simulink model "microgrid_healthy_load_profiling_CDR_revD"  (Simulink 7.9)
settings: Solver=ode3  SolverMode=SingleTasking  StartTime=0.0  StopTime=12  FixedStep=1*10^(-4)  RelTol=1e-3
undefined symbols (not defined in the file): D1, Delta, tl1, tl2, tl3, tl4, tl5, tl6, Ts
libraries: powerlib x104, powerlib_extras x36
(part 1 of 2)
settings Model: Creator=SK  LastModifiedBy=SK
settings SolverCC: ZeroCrossAlgorithm=Adaptive  AlgebraicLoopSolver=LineSearch
settings OptimizationCC: SimCompilerOptimization=On  AccelVerboseBuild=on
settings SFSimCC: SFSimEnableDebug=off  SFSimEcho=off
settings RTWCC: RTWCompilerOptimization=On

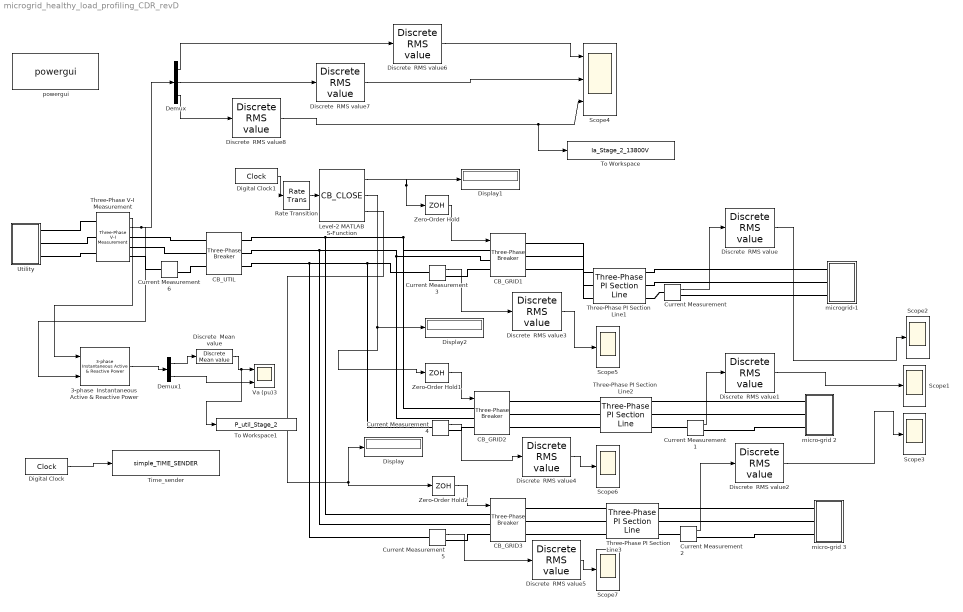
== system microgrid_healthy_load_profiling_CDR_revD ==
  3-phase  Instantaneous  Active & Reactive Power : powerlib_extras/Measurements/3-phase  Instantaneous  Active & Reactive Power
  CB_GRID1 : powerlib/Elements/Three-Phase Breaker  InitialState=closed  SwitchA=on  SwitchB=on  SwitchC=on  SwitchTimes="[4/60  10/60]"  External=on  BreakerResistance=0.001  SnubberResistance=1e6  SnubberCapacitance=inf  Measurements=None
  CB_GRID2 : powerlib/Elements/Three-Phase Breaker  InitialState=closed  SwitchA=on  SwitchB=on  SwitchC=on  SwitchTimes="[4/60  10/60]"  External=on  BreakerResistance=0.001  SnubberResistance=1e6  SnubberCapacitance=inf  Measurements=None
  CB_GRID3 : powerlib/Elements/Three-Phase Breaker  InitialState=closed  SwitchA=on  SwitchB=on  SwitchC=on  SwitchTimes="[4/60  10/60]"  External=on  BreakerResistance=0.001  SnubberResistance=1e6  SnubberCapacitance=inf  Measurements=None
  CB_UTIL : powerlib/Elements/Three-Phase Breaker  InitialState=closed  SwitchA=off  SwitchB=off  SwitchC=off  SwitchTimes="[4/60  10/60]"  External=off  BreakerResistance=0.001  SnubberResistance=1e6  SnubberCapacitance=inf  Measurements=None
  Current Measurement{,1..6} (7 alike) : powerlib/Measurements/Current Measurement  PhasorSimulation=off  OutputType=Complex  PSBequivalent=0
  Demux : Demux  Outputs=3
  Demux1 : Demux  Outputs=2
  Digital Clock : DigitalClock  SampleTime=Ts
  Digital Clock1 : DigitalClock  SampleTime=1e-4
  Discrete  Mean value : powerlib_extras/Discrete Measurements/Discrete  Mean value  Freq=60  Vinit=0  Ts=Ts
  Discrete  RMS value{,1..8} (9 alike) : powerlib_extras/Discrete Measurements/Discrete  RMS value  Freq=60  Mag_Init=0  Ts=Ts
  Display : Display
  Display1 : Display
  Display2 : Display
  Level-2 MATLAB S-Function : M-S-Function  FunctionName=CB_CLOSE
  Rate Transition : RateTransition
  Scope{1..3,5..7} (6 alike) : Scope
      Scope1 settings: YMin=0.95  YMax=1.05  SaveName=ScopeData3
      Scope2 settings: TimeRange=12  YMin=0  YMax=90
      Scope3 settings: YMin=0.95  YMax=1.05  SaveName=ScopeData4
      Scope5 settings: TimeRange=12  YMin=0  YMax=90  SaveName=ScopeData19
      Scope6 settings: TimeRange=12  YMin=0  YMax=90  SaveName=ScopeData20
      Scope7 settings: TimeRange=12  YMin=0  YMax=90  SaveName=ScopeData21
  Scope4 : Scope  NumInputPorts=3
      settings: TimeRange=12  YMin=54.0598~54.0598~54.0598  YMax=59.7504~59.7504~59.7504
  Three-Phase PI Section Line1 : powerlib/Elements/Three-Phase PI Section Line  LConnTagsString=a|b|c  RConnTagsString=A|B|C  Frequency=60  Resistances=[ 36.757 0.0]  Inductances="[ 0.126  0.0001]"  Capacitances=[0.00001 0.0001]  Length=2.06
  Three-Phase PI Section Line2 : powerlib/Elements/Three-Phase PI Section Line  LConnTagsString=a|b|c  RConnTagsString=A|B|C  Frequency=60  Resistances=[ 36.757 0.0]  Inductances="[ 0.126  0.0001]"  Capacitances=[0.00001 0.0001]  Length=2.06
  Three-Phase PI Section Line3 : powerlib/Elements/Three-Phase PI Section Line  LConnTagsString=a|b|c  RConnTagsString=A|B|C  Frequency=60  Resistances=[ 36.757 0.0]  Inductances="[ 0.126  0.0001]"  Capacitances=[0.00001 0.0001]  Length=2.06
  Three-Phase V-I Measurement : powerlib/Measurements/Three-Phase V-I Measurement  VoltageMeasurement=phase-to-ground  SetLabelV=off  LabelV=Vabc  Vpu=off  VpuLL=off  CurrentMeasurement=yes  SetLabelI=off  LabelI=Iabc  Ipu=off  Pbase=100e6  Vbase=500e3  OutputType=Magnitude  PhasorSimulation=off  PSBequivalent=0
  Time_sender : M-S-Function  FunctionName=simple_TIME_SENDER
  To Workspace : ToWorkspace  VariableName=Ia_Stage_2_13800V  SampleTime=5*Ts  SaveFormat=Structure With Time
  To Workspace1 : ToWorkspace  VariableName=P_util_Stage_2  SampleTime=5*Ts
  Utility : Subsystem
  Va (pu)3 : Scope  NumInputPorts=2
      settings: TickLabels=on  TimeRange=2  YMin=882000~-447440  YMax=974842~-447345  SaveName=vf
  Zero-Order Hold : ZeroOrderHold  SampleTime=0.3
  Zero-Order Hold1 : ZeroOrderHold  SampleTime=0.3
  Zero-Order Hold2 : ZeroOrderHold  SampleTime=0.3
  micro-grid 2 : Subsystem
  micro-grid 3 : Subsystem
  microgrid-1 : Subsystem
  powergui : powerlib/powergui  Priority=1  SimulationMode=Discrete  SolverType=Tustin  SampleTime=Ts  frequency=60  SPID=on  DisableSnubberDevices=off  DisableRonSwitches=off  DisableVfSwitches=off  SwTol=0  Interpol=off  DisplayEquations=off  FunctionMessages=off  frequencyindice=60  Pbase=5e6  ErrMax=1e-4  Iterations=50  UnitsV=kV  UnitsW=MW  echomessages=off  HookPort=off  EnableUseOfTLC=off  x0status=blocks  RestoreLinks=warning  ResistiveCurrentMeasurement=off  Ylog=off  Xlog=on  ShowGrid=off  save=off  variable=ZData  structure=y  ZoomFFT=off  StartTime=0.0  cycles=1  DisplayStyle=1  fundamental=60  FreqAxis=off  MaxFrequency=1000  frequencyindicesteady=1  display=off  methode=off
  wires:
  Zero-Order Hold/1 -> CB_GRID1/1
  Digital Clock/1 -> Time_sender/1
  Digital Clock1/1 -> Rate Transition/1
  Rate Transition/1 -> Level-2 MATLAB S-Function/1
  Zero-Order Hold1/1 -> CB_GRID2/1
  Zero-Order Hold2/1 -> CB_GRID3/1
  Level-2 MATLAB S-Function/1 -> Zero-Order Hold/1, Display1/1
  Level-2 MATLAB S-Function/2 -> Zero-Order Hold1/1, Display2/1
  Level-2 MATLAB S-Function/3 -> Zero-Order Hold2/1, Display/1
  Current Measurement/1 -> Discrete  RMS value/1
  Current Measurement1/1 -> Discrete  RMS value1/1
  Current Measurement2/1 -> Discrete  RMS value2/1
  Discrete  RMS value/1 -> Scope2/1
  Discrete  RMS value1/1 -> Scope1/1
  Discrete  RMS value2/1 -> Scope3/1
  Current Measurement3/1 -> Discrete  RMS value3/1
  Discrete  RMS value3/1 -> Scope5/1
  Current Measurement4/1 -> Discrete  RMS value4/1
  Discrete  RMS value4/1 -> Scope6/1
  Current Measurement5/1 -> Discrete  RMS value5/1
  Discrete  RMS value5/1 -> Scope7/1
  Three-Phase V-I Measurement/2 -> Demux/1, 3-phase  Instantaneous  Active & Reactive Power/2
  Demux/1 -> Discrete  RMS value6/1
  Demux/2 -> Discrete  RMS value7/1
  Demux/3 -> Discrete  RMS value8/1
  Discrete  RMS value6/1 -> Scope4/1
  Discrete  RMS value7/1 -> Scope4/2
  Discrete  RMS value8/1 -> Scope4/3, To Workspace/1
  Demux1/2 -> Va (pu)3/2
  Three-Phase V-I Measurement/1 -> 3-phase  Instantaneous  Active & Reactive Power/1
  3-phase  Instantaneous  Active & Reactive Power/1 -> Demux1/1
  Demux1/1 -> Discrete  Mean value/1
  Discrete  Mean value/1 -> Va (pu)3/1, To Workspace1/1
  connections:
  Three-Phase V-I Measurement/RConn2 -- CB_UTIL/LConn2
  Utility/RConn2 -- Three-Phase V-I Measurement/LConn2
  Three-Phase V-I Measurement/RConn1 -- CB_UTIL/LConn1
  Utility/RConn1 -- Three-Phase V-I Measurement/LConn1
  Three-Phase V-I Measurement/LConn3 -- Utility/RConn3
  CB_UTIL/RConn1 -- CB_GRID2/LConn1 -- CB_GRID1/LConn1 -- CB_GRID3/LConn1
  CB_UTIL/RConn2 -- CB_GRID2/LConn2 -- CB_GRID1/LConn2 -- CB_GRID3/LConn2
  Current Measurement3/LConn1 -- Current Measurement4/LConn1 -- CB_UTIL/RConn3 -- Current Measurement5/LConn1
  Three-Phase PI Section Line3/RConn1 -- micro-grid 3/LConn1
  Three-Phase PI Section Line3/RConn2 -- micro-grid 3/LConn2
  Three-Phase PI Section Line1/RConn1 -- microgrid-1/LConn1
  Three-Phase PI Section Line1/RConn2 -- microgrid-1/LConn2
  Three-Phase PI Section Line2/RConn1 -- micro-grid 2/LConn1
  Three-Phase PI Section Line2/RConn2 -- micro-grid 2/LConn2
  CB_GRID3/RConn1 -- Three-Phase PI Section Line3/LConn1
  CB_GRID3/RConn2 -- Three-Phase PI Section Line3/LConn2
  CB_GRID2/RConn1 -- Three-Phase PI Section Line2/LConn1
  CB_GRID2/RConn2 -- Three-Phase PI Section Line2/LConn2
  CB_GRID1/RConn1 -- Three-Phase PI Section Line1/LConn1
  CB_GRID1/RConn2 -- Three-Phase PI Section Line1/LConn2
  CB_GRID1/RConn3 -- Three-Phase PI Section Line1/LConn3
  Three-Phase PI Section Line1/RConn3 -- Current Measurement/LConn1
  Current Measurement/RConn1 -- microgrid-1/LConn3
  Three-Phase PI Section Line2/RConn3 -- Current Measurement1/LConn1
  Current Measurement1/RConn1 -- micro-grid 2/LConn3
  Three-Phase PI Section Line3/RConn3 -- Current Measurement2/LConn1
  Current Measurement2/RConn1 -- micro-grid 3/LConn3
  CB_GRID3/RConn3 -- Three-Phase PI Section Line3/LConn3
  CB_GRID2/RConn3 -- Three-Phase PI Section Line2/LConn3
  Current Measurement3/RConn1 -- CB_GRID1/LConn3
  Current Measurement4/RConn1 -- CB_GRID2/LConn3
  Current Measurement5/RConn1 -- CB_GRID3/LConn3
  Three-Phase V-I Measurement/RConn3 -- Current Measurement6/LConn1
  Current Measurement6/RConn1 -- CB_UTIL/LConn3

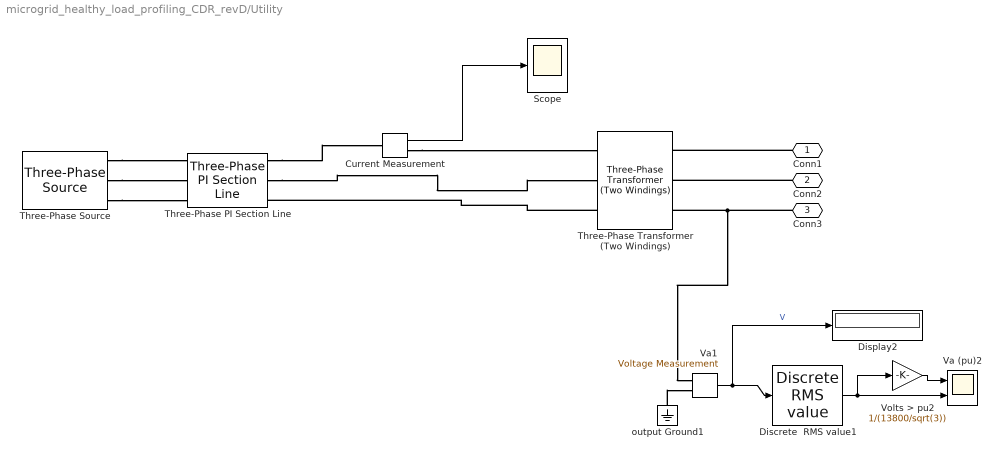
== system microgrid_healthy_load_profiling_CDR_revD/Utility ==
  Current Measurement : powerlib/Measurements/Current Measurement  PhasorSimulation=off  OutputType=Complex  PSBequivalent=0
  Discrete  RMS value1 : powerlib_extras/Discrete Measurements/Discrete  RMS value  Freq=60  Mag_Init=0  Ts=Ts
  Display2 : Display
  Scope : Scope
      settings: YMin=-17.5  YMax=17.5  SaveName=ScopeData2
  Three-Phase PI Section Line : powerlib/Elements/Three-Phase PI Section Line  LConnTagsString=a|b|c  RConnTagsString=A|B|C  Frequency=60  Resistances=[ 0.9428 0.0]  Inductances="[ 4.9e-3  0.00001]"  Capacitances=[0.00001 0.0001]  Length=3.05
  Three-Phase Transformer (Two Windings) : powerlib/Elements/Three-Phase Transformer (Two Windings)  Winding1Connection=Delta (D1)  UNITS=pu  NominalPower=[ 15e6 , 60 ]  Winding1=[ 69e3 , 0.667 , 5.33 ]  Winding2Connection=Yg  Winding2=[ 13.8e3 , 0.667 , 5.33 ]  SetSaturation=off  Rm=500  Lm=500  Saturation=[ 0,0 ; 0.0024,1.2 ; 1.0,1.52 ]  Hysteresis=off  DataFile='hysteresis'  SetInitialFlux=off  InitialFluxes=[ 0.8 , -0.8 , 0.7 ]  Measurements=None  MoreParameters=off  BreakLoop=off  DataType=off  TransfoNumber=1
  Three-Phase Source : powerlib/Electrical Sources/Three-Phase Source  Voltage=69e3  PhaseAngle=0  Frequency=60  InternalConnection=Yg  SpecifyImpedance=on  Resistance=0.8929  Inductance=16.58e-3  ShortCircuitLevel=10000e6  BaseVoltage=69e3  XRratio=22.2  BusType=swing  Pref=0  Qref=0  Qmin=-inf  Qmax=inf
  Va (pu)2 : Scope  NumInputPorts=2
      settings: TickLabels=on  TimeRange=3  YMin=1.2931~10302  YMax=1.2946~10315  SaveName=vf1
  Va1 : powerlib/Measurements/Voltage Measurement  Tag=PoWeRsYsTeMmEaSuReMeNt  PhasorSimulation=off  OutputType=Magnitude  PSBequivalent=0
  Volts > pu2 : Gain  Gain=1/(13800/sqrt(3))  SaturateOnIntegerOverflow=on  OutDataTypeStr=Inherit: Same as input  ParamDataTypeStr=Inherit: Same as input
  output Ground1 : powerlib/Elements/Ground  LConnTagsString=a
  Conn1 : PMIOPort  Port=1  Side=Right
  Conn2 : PMIOPort  Port=2  Side=Right
  Conn3 : PMIOPort  Port=3  Side=Right
  wires:
  Va1/1 -> Discrete  RMS value1/1, Display2/1  "V"
  Discrete  RMS value1/1 -> Va (pu)2/2, Volts > pu2/1
  Volts > pu2/1 -> Va (pu)2/1
  Current Measurement/1 -> Scope/1
  connections:
  Three-Phase Source/RConn1 -- Three-Phase PI Section Line/RConn1
  Three-Phase Source/RConn2 -- Three-Phase PI Section Line/RConn2
  Three-Phase Source/RConn3 -- Three-Phase PI Section Line/RConn3
  Conn1/RConn1 -- Three-Phase Transformer (Two Windings)/RConn1
  Conn2/RConn1 -- Three-Phase Transformer (Two Windings)/RConn2
  Conn3/RConn1 -- Three-Phase Transformer (Two Windings)/RConn3 -- Va1/LConn1
  Three-Phase PI Section Line/LConn2 -- Three-Phase Transformer (Two Windings)/LConn2
  Three-Phase Transformer (Two Windings)/LConn3 -- Three-Phase PI Section Line/LConn3
  output Ground1/LConn1 -- Va1/LConn2
  Three-Phase PI Section Line/LConn1 -- Current Measurement/LConn1
  Current Measurement/RConn1 -- Three-Phase Transformer (Two Windings)/LConn1

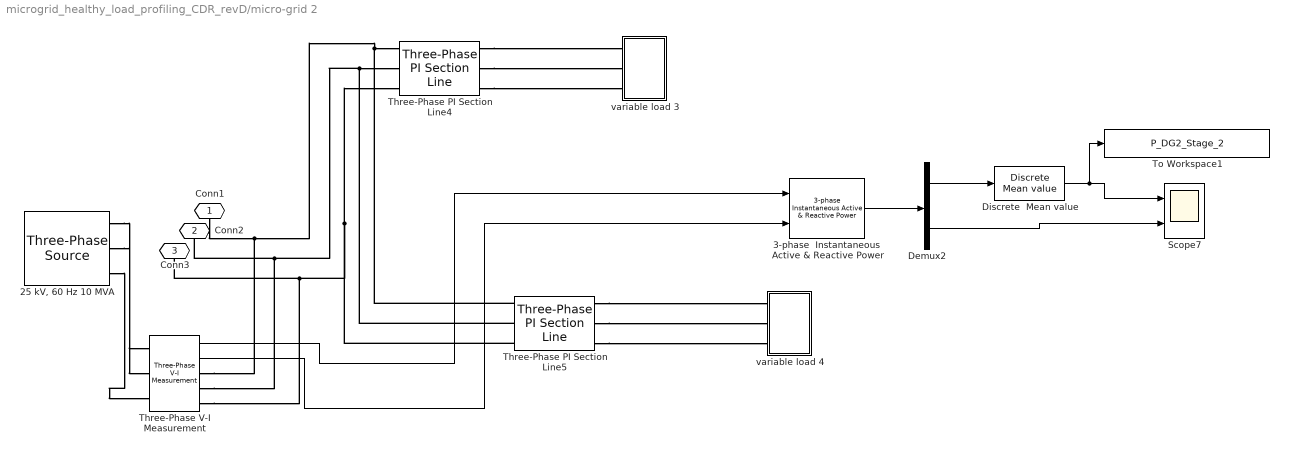
== system microgrid_healthy_load_profiling_CDR_revD/micro-grid 2 ==
  "25 kV, 60 Hz 10 MVA" : powerlib/Electrical Sources/Three-Phase Source  Voltage=13.8e3  PhaseAngle=0  Frequency=60  InternalConnection=Yg  SpecifyImpedance=on  Resistance=25e3^2/10e6/5  Inductance=25e3^2/10e6/377  ShortCircuitLevel=22.72e6  BaseVoltage=13.8e3  XRratio=0.75  BusType=PV  Pref=4e6  Qref=0  Qmin=-inf  Qmax=inf
  3-phase  Instantaneous  Active & Reactive Power : powerlib_extras/Measurements/3-phase  Instantaneous  Active & Reactive Power
  Demux2 : Demux  Outputs=2
  Discrete  Mean value : powerlib_extras/Discrete Measurements/Discrete  Mean value  Freq=60  Vinit=0  Ts=Ts
  Scope7 : Scope  NumInputPorts=2
      settings: YMin=85.375~88.91  YMax=85.625~89.03  SaveName=ScopeData14
  Three-Phase PI Section Line4 : powerlib/Elements/Three-Phase PI Section Line  LConnTagsString=a|b|c  RConnTagsString=A|B|C  Frequency=60  Resistances=[13.8 0.0]  Inductances="[ 0.046  0.0001]"  Capacitances=[0.00001 0.0001]  Length=0.148
  Three-Phase PI Section Line5 : powerlib/Elements/Three-Phase PI Section Line  LConnTagsString=a|b|c  RConnTagsString=A|B|C  Frequency=60  Resistances=[ 134.04 0.0]  Inductances="[ 0.046  0.0001]"  Capacitances=[0.00001 0.0001]  Length=0.104
  Three-Phase V-I Measurement : powerlib/Measurements/Three-Phase V-I Measurement  VoltageMeasurement=phase-to-ground  SetLabelV=off  LabelV=Vabc  Vpu=off  VpuLL=off  CurrentMeasurement=yes  SetLabelI=off  LabelI=Iabc  Ipu=off  Pbase=100e6  Vbase=500e3  OutputType=Magnitude  PhasorSimulation=off  PSBequivalent=0
  To Workspace1 : ToWorkspace  VariableName=P_DG2_Stage_2  SampleTime=5*Ts
  variable load 3 : Subsystem
  variable load 4 : Subsystem
  Conn1 : PMIOPort  Port=1  Side=Left
  Conn2 : PMIOPort  Port=2  Side=Left
  Conn3 : PMIOPort  Port=3  Side=Left
  wires:
  Three-Phase V-I Measurement/1 -> 3-phase  Instantaneous  Active & Reactive Power/1
  Three-Phase V-I Measurement/2 -> 3-phase  Instantaneous  Active & Reactive Power/2
  3-phase  Instantaneous  Active & Reactive Power/1 -> Demux2/1
  Demux2/1 -> Discrete  Mean value/1
  Discrete  Mean value/1 -> Scope7/1, To Workspace1/1
  Demux2/2 -> Scope7/2
  connections:
  Three-Phase PI Section Line4/LConn3 -- Three-Phase PI Section Line5/LConn3 -- Conn3/RConn1 -- Three-Phase V-I Measurement/RConn3
  Three-Phase PI Section Line4/LConn2 -- Three-Phase PI Section Line5/LConn2 -- Conn2/RConn1 -- Three-Phase V-I Measurement/RConn2
  Conn1/RConn1 -- Three-Phase PI Section Line4/LConn1 -- Three-Phase PI Section Line5/LConn1 -- Three-Phase V-I Measurement/RConn1
  Three-Phase PI Section Line4/RConn1 -- variable load 3/LConn1
  Three-Phase PI Section Line4/RConn2 -- variable load 3/LConn2
  Three-Phase PI Section Line4/RConn3 -- variable load 3/LConn3
  Three-Phase PI Section Line5/RConn1 -- variable load 4/LConn1
  Three-Phase PI Section Line5/RConn2 -- variable load 4/LConn2
  Three-Phase PI Section Line5/RConn3 -- variable load 4/LConn3
  "25 kV, 60 Hz 10 MVA"/RConn1 -- Three-Phase V-I Measurement/LConn1
  "25 kV, 60 Hz 10 MVA"/RConn2 -- Three-Phase V-I Measurement/LConn2
  "25 kV, 60 Hz 10 MVA"/RConn3 -- Three-Phase V-I Measurement/LConn3

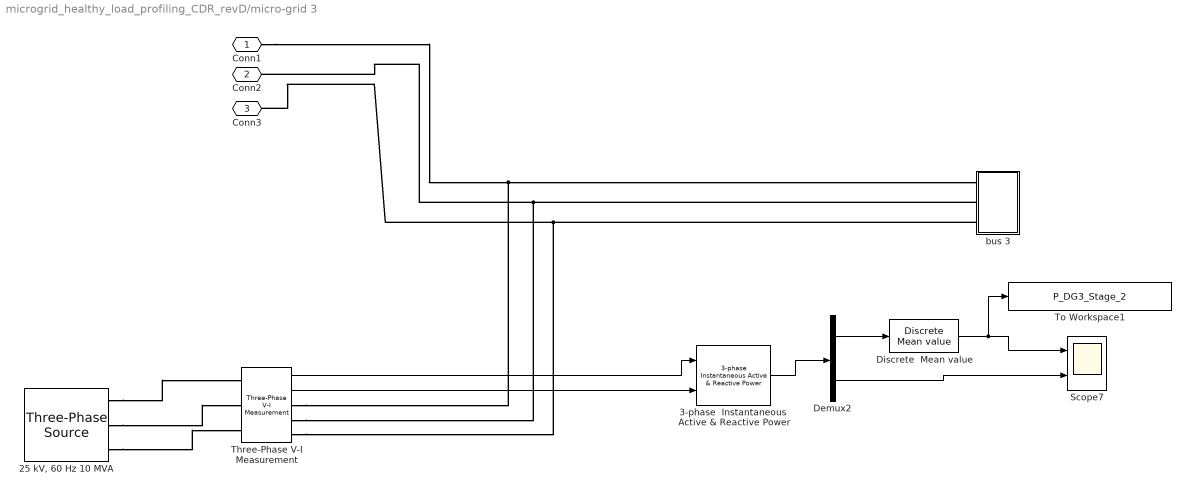
== system microgrid_healthy_load_profiling_CDR_revD/micro-grid 3 ==
  "25 kV, 60 Hz 10 MVA" : powerlib/Electrical Sources/Three-Phase Source  Voltage=13.8e3  PhaseAngle=0  Frequency=60  InternalConnection=Yg  SpecifyImpedance=on  Resistance=25e3^2/10e6/5  Inductance=25e3^2/10e6/377  ShortCircuitLevel=16.67e6  BaseVoltage=13.8e3  XRratio=0.75  BusType=PV  Pref=2e6  Qref=0  Qmin=-inf  Qmax=inf
  3-phase  Instantaneous  Active & Reactive Power : powerlib_extras/Measurements/3-phase  Instantaneous  Active & Reactive Power
  Demux2 : Demux  Outputs=2
  Discrete  Mean value : powerlib_extras/Discrete Measurements/Discrete  Mean value  Freq=60  Vinit=0  Ts=Ts
  Scope7 : Scope  NumInputPorts=2
      settings: YMin=85.375~88.91  YMax=85.625~89.03  SaveName=ScopeData22
  Three-Phase V-I Measurement : powerlib/Measurements/Three-Phase V-I Measurement  VoltageMeasurement=phase-to-ground  SetLabelV=off  LabelV=Vabc  Vpu=off  VpuLL=off  CurrentMeasurement=yes  SetLabelI=off  LabelI=Iabc  Ipu=off  Pbase=100e6  Vbase=500e3  OutputType=Magnitude  PhasorSimulation=off  PSBequivalent=0
  To Workspace1 : ToWorkspace  VariableName=P_DG3_Stage_2  SampleTime=5*Ts
  bus 3 : Subsystem
  Conn1 : PMIOPort  Port=1  Side=Left
  Conn2 : PMIOPort  Port=2  Side=Left
  Conn3 : PMIOPort  Port=3  Side=Left
  wires:
  Three-Phase V-I Measurement/1 -> 3-phase  Instantaneous  Active & Reactive Power/1
  Three-Phase V-I Measurement/2 -> 3-phase  Instantaneous  Active & Reactive Power/2
  3-phase  Instantaneous  Active & Reactive Power/1 -> Demux2/1
  Demux2/1 -> Discrete  Mean value/1
  Demux2/2 -> Scope7/2
  Discrete  Mean value/1 -> Scope7/1, To Workspace1/1
  connections:
  bus 3/LConn2 -- Conn2/RConn1 -- Three-Phase V-I Measurement/RConn2
  Conn1/RConn1 -- bus 3/LConn1 -- Three-Phase V-I Measurement/RConn1
  bus 3/LConn3 -- Conn3/RConn1 -- Three-Phase V-I Measurement/RConn3
  "25 kV, 60 Hz 10 MVA"/RConn1 -- Three-Phase V-I Measurement/LConn1
  "25 kV, 60 Hz 10 MVA"/RConn2 -- Three-Phase V-I Measurement/LConn2
  "25 kV, 60 Hz 10 MVA"/RConn3 -- Three-Phase V-I Measurement/LConn3

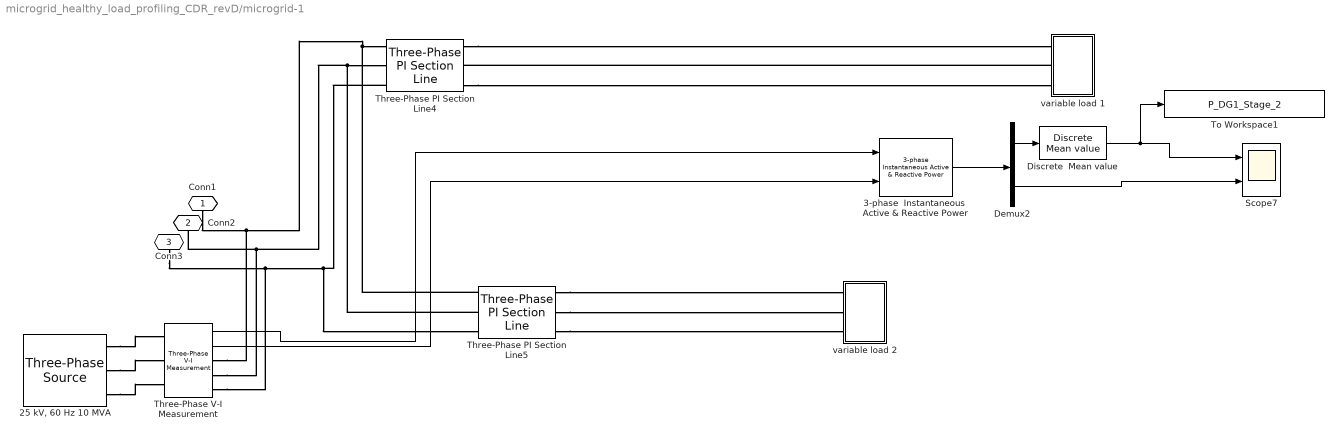
== system microgrid_healthy_load_profiling_CDR_revD/microgrid-1 ==
  "25 kV, 60 Hz 10 MVA" : powerlib/Electrical Sources/Three-Phase Source  Voltage=13.8e3  PhaseAngle=0  Frequency=60  InternalConnection=Yg  SpecifyImpedance=on  Resistance=25e3^2/10e6/5  Inductance=25e3^2/10e6/377  ShortCircuitLevel=22.72e6  BaseVoltage=13.8e3  XRratio=0.75  BusType=PV  Pref=4e6  Qref=0  Qmin=-inf  Qmax=inf
  3-phase  Instantaneous  Active & Reactive Power : powerlib_extras/Measurements/3-phase  Instantaneous  Active & Reactive Power
  Demux2 : Demux  Outputs=2
  Discrete  Mean value : powerlib_extras/Discrete Measurements/Discrete  Mean value  Freq=60  Vinit=0  Ts=Ts
  Scope7 : Scope  NumInputPorts=2
      settings: YMin=85.375~88.91  YMax=85.625~89.03  SaveName=ScopeData9
  Three-Phase PI Section Line4 : powerlib/Elements/Three-Phase PI Section Line  LConnTagsString=a|b|c  RConnTagsString=A|B|C  Frequency=60  Resistances=[13.8 0.0]  Inductances="[ 0.046  0.0001]"  Capacitances=[0.00001 0.0001]  Length=0.148
  Three-Phase PI Section Line5 : powerlib/Elements/Three-Phase PI Section Line  LConnTagsString=a|b|c  RConnTagsString=A|B|C  Frequency=60  Resistances=[ 134.04 0.0]  Inductances="[ 0.046  0.0001]"  Capacitances=[0.00001 0.0001]  Length=0.104
  Three-Phase V-I Measurement : powerlib/Measurements/Three-Phase V-I Measurement  VoltageMeasurement=phase-to-ground  SetLabelV=off  LabelV=Vabc  Vpu=off  VpuLL=off  CurrentMeasurement=yes  SetLabelI=off  LabelI=Iabc  Ipu=off  Pbase=100e6  Vbase=500e3  OutputType=Magnitude  PhasorSimulation=off  PSBequivalent=0
  To Workspace1 : ToWorkspace  VariableName=P_DG1_Stage_2  SampleTime=5*Ts
  variable load 1 : Subsystem
  variable load 2 : Subsystem
  Conn1 : PMIOPort  Port=1  Side=Left
  Conn2 : PMIOPort  Port=2  Side=Left
  Conn3 : PMIOPort  Port=3  Side=Left
  wires:
  Three-Phase V-I Measurement/1 -> 3-phase  Instantaneous  Active & Reactive Power/1
  Three-Phase V-I Measurement/2 -> 3-phase  Instantaneous  Active & Reactive Power/2
  3-phase  Instantaneous  Active & Reactive Power/1 -> Demux2/1
  Demux2/1 -> Discrete  Mean value/1
  Demux2/2 -> Scope7/2
  Discrete  Mean value/1 -> Scope7/1, To Workspace1/1
  connections:
  Conn1/RConn1 -- Three-Phase PI Section Line5/LConn1 -- Three-Phase PI Section Line4/LConn1 -- Three-Phase V-I Measurement/RConn1
  Three-Phase PI Section Line5/LConn2 -- Three-Phase PI Section Line4/LConn2 -- Conn2/RConn1 -- Three-Phase V-I Measurement/RConn2
  Conn3/RConn1 -- Three-Phase PI Section Line4/LConn3 -- Three-Phase PI Section Line5/LConn3 -- Three-Phase V-I Measurement/RConn3
  variable load 1/LConn2 -- Three-Phase PI Section Line4/RConn2
  Three-Phase PI Section Line4/RConn3 -- variable load 1/LConn3
  Three-Phase PI Section Line4/RConn1 -- variable load 1/LConn1
  Three-Phase PI Section Line5/RConn1 -- variable load 2/LConn1
  Three-Phase PI Section Line5/RConn2 -- variable load 2/LConn2
  Three-Phase PI Section Line5/RConn3 -- variable load 2/LConn3
  "25 kV, 60 Hz 10 MVA"/RConn1 -- Three-Phase V-I Measurement/LConn1
  "25 kV, 60 Hz 10 MVA"/RConn2 -- Three-Phase V-I Measurement/LConn2
  "25 kV, 60 Hz 10 MVA"/RConn3 -- Three-Phase V-I Measurement/LConn3

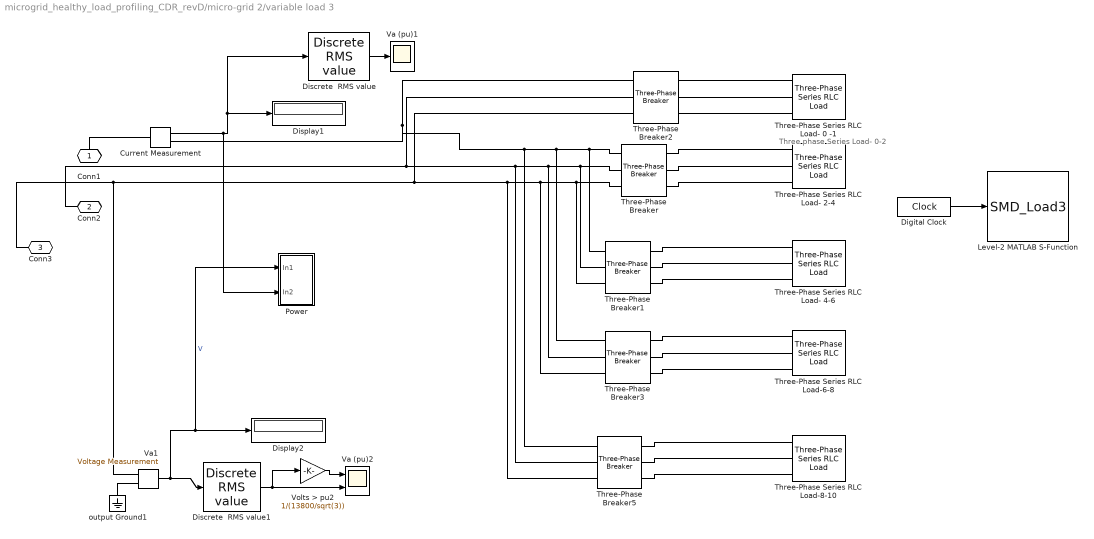
== system microgrid_healthy_load_profiling_CDR_revD/micro-grid 2/variable load 3 ==
  note: Three phase Series Load- 0-2
  Current Measurement : powerlib/Measurements/Current Measurement  PhasorSimulation=off  OutputType=Complex  PSBequivalent=0
  Digital Clock : DigitalClock  SampleTime=Ts
  Discrete  RMS value : powerlib_extras/Discrete Measurements/Discrete  RMS value  Freq=60  Mag_Init=0  Ts=Ts
  Discrete  RMS value1 : powerlib_extras/Discrete Measurements/Discrete  RMS value  Freq=60  Mag_Init=0  Ts=Ts
  Display1 : Display
  Display2 : Display
  Level-2 MATLAB S-Function : M-S-Function  FunctionName=SMD_Load3  Parameters=tl3
  Power : Subsystem
  Three-Phase Series RLC Load- 0 -1 : powerlib/Elements/Three-Phase Series RLC Load  LConnTagsString=A|B|C  Configuration=Y (grounded)  NominalVoltage=13800  NominalFrequency=60  ActivePower=3.64e6  InductivePower=3.43e6  CapacitivePower=0  Measurements=None  LoadType=constant Z
  Three-Phase Series RLC Load- 2-4 : powerlib/Elements/Three-Phase Series RLC Load  LConnTagsString=A|B|C  Configuration=Y (grounded)  NominalVoltage=13800  NominalFrequency=60  ActivePower=4.2e6  InductivePower=0  CapacitivePower=2.71e6  Measurements=None  LoadType=constant Z
  Three-Phase Series RLC Load- 4-6 : powerlib/Elements/Three-Phase Series RLC Load  LConnTagsString=A|B|C  Configuration=Y (grounded)  NominalVoltage=13800  NominalFrequency=60  ActivePower=4e6  InductivePower=3e6  CapacitivePower=0  Measurements=None  LoadType=constant Z
  Three-Phase Series RLC Load-6-8 : powerlib/Elements/Three-Phase Series RLC Load  LConnTagsString=A|B|C  Configuration=Y (grounded)  NominalVoltage=13800  NominalFrequency=60  ActivePower=3.8e6  InductivePower=3.25e6  CapacitivePower=0  Measurements=None  LoadType=constant Z
  Three-Phase Series RLC Load-8-10 : powerlib/Elements/Three-Phase Series RLC Load  LConnTagsString=A|B|C  Configuration=Y (grounded)  NominalVoltage=13800  NominalFrequency=60  ActivePower=3.72e6  InductivePower=3.34e6  CapacitivePower=0  Measurements=None  LoadType=constant Z
  Three-Phase Breaker : powerlib/Elements/Three-Phase Breaker  InitialState=open  SwitchA=on  SwitchB=on  SwitchC=on  SwitchTimes=[tl3(1)/60 tl3(2)/60]  External=off  BreakerResistance=0.001  SnubberResistance=1e6  SnubberCapacitance=inf  Measurements=None
  Three-Phase Breaker1 : powerlib/Elements/Three-Phase Breaker  InitialState=open  SwitchA=on  SwitchB=on  SwitchC=on  SwitchTimes="[tl3(2)/60  tl3(3)/60]"  External=off  BreakerResistance=0.001  SnubberResistance=1e6  SnubberCapacitance=inf  Measurements=None
  Three-Phase Breaker2 : powerlib/Elements/Three-Phase Breaker  InitialState=closed  SwitchA=on  SwitchB=on  SwitchC=on  SwitchTimes=[tl3(1)/60]  External=off  BreakerResistance=0.001  SnubberResistance=1e6  SnubberCapacitance=inf  Measurements=None
  Three-Phase Breaker3 : powerlib/Elements/Three-Phase Breaker  InitialState=open  SwitchA=on  SwitchB=on  SwitchC=on  SwitchTimes="[tl3(3)/60  tl3(4)/60]"  External=off  BreakerResistance=0.001  SnubberResistance=1e6  SnubberCapacitance=inf  Measurements=None
  Three-Phase Breaker5 : powerlib/Elements/Three-Phase Breaker  InitialState=open  SwitchA=on  SwitchB=on  SwitchC=on  SwitchTimes=[tl3(4)/60]  External=off  BreakerResistance=0.001  SnubberResistance=1e6  SnubberCapacitance=inf  Measurements=None
  Va (pu)1 : Scope
      settings: TickLabels=on  TimeRange=2  YMin=-0.8  YMax=0.8  SaveName=vf6
  Va (pu)2 : Scope  NumInputPorts=2
      settings: TickLabels=on  TimeRange=3  YMin=0.8979~7153.5  YMax=0.8991~7163.5  SaveName=vf2
  Va1 : powerlib/Measurements/Voltage Measurement  Tag=PoWeRsYsTeMmEaSuReMeNt  PhasorSimulation=off  OutputType=Magnitude  PSBequivalent=0
  Volts > pu2 : Gain  Gain=1/(13800/sqrt(3))  SaturateOnIntegerOverflow=on  OutDataTypeStr=Inherit: Same as input  ParamDataTypeStr=Inherit: Same as input
  output Ground1 : powerlib/Elements/Ground  LConnTagsString=a
  Conn1 : PMIOPort  Port=1  Side=Left
  Conn2 : PMIOPort  Port=2  Side=Left
  Conn3 : PMIOPort  Port=3  Side=Left
  wires:
  Volts > pu2/1 -> Va (pu)2/1
  Discrete  RMS value1/1 -> Volts > pu2/1, Va (pu)2/2
  Discrete  RMS value/1 -> Va (pu)1/1
  Current Measurement/1 -> Power/2(In2), Display1/1, Discrete  RMS value/1
  Va1/1 -> Discrete  RMS value1/1, Power/1(In1), Display2/1  "V"
  Digital Clock/1 -> Level-2 MATLAB S-Function/1
  connections:
  Three-Phase Breaker5/RConn3 -- Three-Phase Series RLC Load-8-10/LConn3
  Three-Phase Breaker5/RConn2 -- Three-Phase Series RLC Load-8-10/LConn2
  Three-Phase Breaker5/RConn1 -- Three-Phase Series RLC Load-8-10/LConn1
  Three-Phase Breaker3/RConn3 -- Three-Phase Series RLC Load-6-8/LConn3
  Three-Phase Breaker3/RConn2 -- Three-Phase Series RLC Load-6-8/LConn2
  Three-Phase Breaker3/RConn1 -- Three-Phase Series RLC Load-6-8/LConn1
  Three-Phase Breaker2/RConn1 -- Three-Phase Series RLC Load- 0 -1/LConn1
  Conn1/RConn1 -- Current Measurement/LConn1
  output Ground1/LConn1 -- Va1/LConn2
  Three-Phase Breaker2/RConn3 -- Three-Phase Series RLC Load- 0 -1/LConn3
  Three-Phase Breaker2/RConn2 -- Three-Phase Series RLC Load- 0 -1/LConn2
  Three-Phase Breaker3/LConn3 -- Three-Phase Breaker1/LConn3 -- Three-Phase Breaker/LConn3 -- Three-Phase Breaker2/LConn3 -- Va1/LConn1 -- Conn3/RConn1 -- Three-Phase Breaker5/LConn3
  Three-Phase Breaker3/LConn2 -- Three-Phase Breaker1/LConn2 -- Three-Phase Breaker/LConn2 -- Three-Phase Breaker2/LConn2 -- Conn2/RConn1 -- Three-Phase Breaker5/LConn2
  Three-Phase Breaker3/LConn1 -- Three-Phase Breaker1/LConn1 -- Three-Phase Breaker/LConn1 -- Three-Phase Breaker2/LConn1 -- Current Measurement/RConn1 -- Three-Phase Breaker5/LConn1
  Three-Phase Breaker1/RConn3 -- Three-Phase Series RLC Load- 4-6/LConn3
  Three-Phase Breaker1/RConn2 -- Three-Phase Series RLC Load- 4-6/LConn2
  Three-Phase Breaker1/RConn1 -- Three-Phase Series RLC Load- 4-6/LConn1
  Three-Phase Breaker/RConn3 -- Three-Phase Series RLC Load- 2-4/LConn3
  Three-Phase Breaker/RConn2 -- Three-Phase Series RLC Load- 2-4/LConn2
  Three-Phase Breaker/RConn1 -- Three-Phase Series RLC Load- 2-4/LConn1

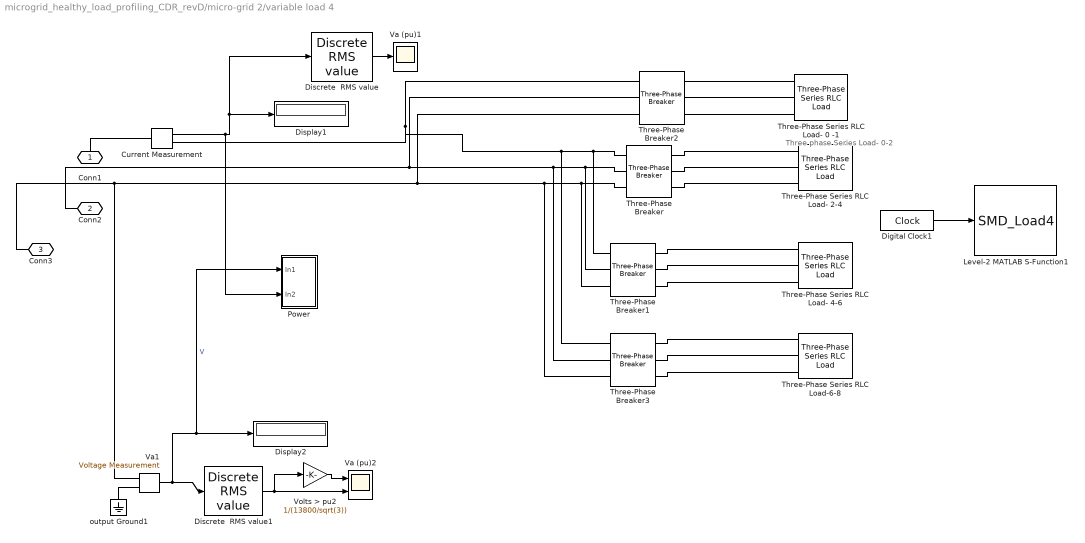
== system microgrid_healthy_load_profiling_CDR_revD/micro-grid 2/variable load 4 ==
  note: Three phase Series Load- 0-2
  Current Measurement : powerlib/Measurements/Current Measurement  PhasorSimulation=off  OutputType=Complex  PSBequivalent=0
  Digital Clock1 : DigitalClock  SampleTime=Ts
  Discrete  RMS value : powerlib_extras/Discrete Measurements/Discrete  RMS value  Freq=60  Mag_Init=0  Ts=Ts
  Discrete  RMS value1 : powerlib_extras/Discrete Measurements/Discrete  RMS value  Freq=60  Mag_Init=0  Ts=Ts
  Display1 : Display
  Display2 : Display
  Level-2 MATLAB S-Function1 : M-S-Function  FunctionName=SMD_Load4  Parameters=tl4
  Power : Subsystem
  Three-Phase Series RLC Load- 0 -1 : powerlib/Elements/Three-Phase Series RLC Load  LConnTagsString=A|B|C  Configuration=Y (grounded)  NominalVoltage=13800  NominalFrequency=60  ActivePower=3.95e6  InductivePower=3.065e6  CapacitivePower=0  Measurements=None  LoadType=constant Z
  Three-Phase Series RLC Load- 2-4 : powerlib/Elements/Three-Phase Series RLC Load  LConnTagsString=A|B|C  Configuration=Y (grounded)  NominalVoltage=13800  NominalFrequency=60  ActivePower=3.75e6  InductivePower=0  CapacitivePower=3.3e6  Measurements=None  LoadType=constant Z
  Three-Phase Series RLC Load- 4-6 : powerlib/Elements/Three-Phase Series RLC Load  LConnTagsString=A|B|C  Configuration=Y (grounded)  NominalVoltage=13800  NominalFrequency=60  ActivePower=3.64e6  InductivePower=0  CapacitivePower=3.428e6  Measurements=None  LoadType=constant Z
  Three-Phase Series RLC Load-6-8 : powerlib/Elements/Three-Phase Series RLC Load  LConnTagsString=A|B|C  Configuration=Y (grounded)  NominalVoltage=13800  NominalFrequency=60  ActivePower=4e6  InductivePower=3e6  CapacitivePower=0  Measurements=None  LoadType=constant Z
  Three-Phase Breaker : powerlib/Elements/Three-Phase Breaker  InitialState=open  SwitchA=on  SwitchB=on  SwitchC=on  SwitchTimes="[tl4(1)/60  tl4(2)/60]"  External=off  BreakerResistance=0.001  SnubberResistance=1e6  SnubberCapacitance=inf  Measurements=None
  Three-Phase Breaker1 : powerlib/Elements/Three-Phase Breaker  InitialState=open  SwitchA=on  SwitchB=on  SwitchC=on  SwitchTimes="[tl4(2)/60  tl4(3)/60]"  External=off  BreakerResistance=0.001  SnubberResistance=1e6  SnubberCapacitance=inf  Measurements=None
  Three-Phase Breaker2 : powerlib/Elements/Three-Phase Breaker  InitialState=closed  SwitchA=on  SwitchB=on  SwitchC=on  SwitchTimes=[tl4(1)/60]  External=off  BreakerResistance=0.001  SnubberResistance=1e6  SnubberCapacitance=inf  Measurements=None
  Three-Phase Breaker3 : powerlib/Elements/Three-Phase Breaker  InitialState=open  SwitchA=on  SwitchB=on  SwitchC=on  SwitchTimes=[tl4(3)/60]  External=off  BreakerResistance=0.001  SnubberResistance=1e6  SnubberCapacitance=inf  Measurements=None
  Va (pu)1 : Scope
      settings: TickLabels=on  TimeRange=2  YMin=-0.8  YMax=0.8  SaveName=vf6
  Va (pu)2 : Scope  NumInputPorts=2
      settings: TickLabels=on  TimeRange=3  YMin=0.8979~7153.5  YMax=0.8991~7163.5  SaveName=vf2
  Va1 : powerlib/Measurements/Voltage Measurement  Tag=PoWeRsYsTeMmEaSuReMeNt  PhasorSimulation=off  OutputType=Magnitude  PSBequivalent=0
  Volts > pu2 : Gain  Gain=1/(13800/sqrt(3))  SaturateOnIntegerOverflow=on  OutDataTypeStr=Inherit: Same as input  ParamDataTypeStr=Inherit: Same as input
  output Ground1 : powerlib/Elements/Ground  LConnTagsString=a
  Conn1 : PMIOPort  Port=1  Side=Left
  Conn2 : PMIOPort  Port=2  Side=Left
  Conn3 : PMIOPort  Port=3  Side=Left
  wires:
  Va1/1 -> Display2/1, Power/1(In1), Discrete  RMS value1/1  "V"
  Current Measurement/1 -> Display1/1, Discrete  RMS value/1, Power/2(In2)
  Discrete  RMS value/1 -> Va (pu)1/1
  Discrete  RMS value1/1 -> Va (pu)2/2, Volts > pu2/1
  Volts > pu2/1 -> Va (pu)2/1
  Digital Clock1/1 -> Level-2 MATLAB S-Function1/1
  connections:
  Three-Phase Breaker/RConn1 -- Three-Phase Series RLC Load- 2-4/LConn1
  Three-Phase Breaker/RConn2 -- Three-Phase Series RLC Load- 2-4/LConn2
  Three-Phase Breaker/RConn3 -- Three-Phase Series RLC Load- 2-4/LConn3
  Three-Phase Breaker1/RConn1 -- Three-Phase Series RLC Load- 4-6/LConn1
  Three-Phase Breaker1/RConn2 -- Three-Phase Series RLC Load- 4-6/LConn2
  Three-Phase Breaker1/RConn3 -- Three-Phase Series RLC Load- 4-6/LConn3
  Three-Phase Breaker3/LConn1 -- Current Measurement/RConn1 -- Three-Phase Breaker2/LConn1 -- Three-Phase Breaker/LConn1 -- Three-Phase Breaker1/LConn1
  Three-Phase Breaker3/LConn2 -- Conn2/RConn1 -- Three-Phase Breaker2/LConn2 -- Three-Phase Breaker/LConn2 -- Three-Phase Breaker1/LConn2
  Three-Phase Breaker3/LConn3 -- Conn3/RConn1 -- Va1/LConn1 -- Three-Phase Breaker2/LConn3 -- Three-Phase Breaker/LConn3 -- Three-Phase Breaker1/LConn3
  Three-Phase Breaker2/RConn2 -- Three-Phase Series RLC Load- 0 -1/LConn2
  Three-Phase Breaker2/RConn3 -- Three-Phase Series RLC Load- 0 -1/LConn3
  output Ground1/LConn1 -- Va1/LConn2
  Conn1/RConn1 -- Current Measurement/LConn1
  Three-Phase Breaker2/RConn1 -- Three-Phase Series RLC Load- 0 -1/LConn1
  Three-Phase Breaker3/RConn1 -- Three-Phase Series RLC Load-6-8/LConn1
  Three-Phase Breaker3/RConn2 -- Three-Phase Series RLC Load-6-8/LConn2
  Three-Phase Breaker3/RConn3 -- Three-Phase Series RLC Load-6-8/LConn3

== system microgrid_healthy_load_profiling_CDR_revD/micro-grid 3/bus 3 ==
  Three-Phase PI Section Line1 : powerlib/Elements/Three-Phase PI Section Line  LConnTagsString=a|b|c  RConnTagsString=A|B|C  Frequency=60  Resistances=[13.8 0.0]  Inductances="[ 0.046  0.0001]"  Capacitances=[0.00001 0.0001]  Length=0.148
  Three-Phase PI Section Line2 : powerlib/Elements/Three-Phase PI Section Line  LConnTagsString=a|b|c  RConnTagsString=A|B|C  Frequency=60  Resistances=[ 134.04 0.0]  Inductances="[ 0.046  0.0001]"  Capacitances=[0.00001 0.0001]  Length=0.104
  variable load 5 : Subsystem
  variable load 6 : Subsystem
  Conn1 : PMIOPort  Port=1  Side=Left
  Conn2 : PMIOPort  Port=2  Side=Left
  Conn3 : PMIOPort  Port=3  Side=Left
  connections:
  Three-Phase PI Section Line2/LConn1 -- Conn1/RConn1 -- Three-Phase PI Section Line1/LConn1
  Three-Phase PI Section Line2/LConn2 -- Conn2/RConn1 -- Three-Phase PI Section Line1/LConn2
  Three-Phase PI Section Line2/LConn3 -- Conn3/RConn1 -- Three-Phase PI Section Line1/LConn3
  Three-Phase PI Section Line1/RConn1 -- variable load 5/LConn1
  Three-Phase PI Section Line1/RConn2 -- variable load 5/LConn2
  Three-Phase PI Section Line1/RConn3 -- variable load 5/LConn3
  Three-Phase PI Section Line2/RConn1 -- variable load 6/LConn1
  Three-Phase PI Section Line2/RConn2 -- variable load 6/LConn2
  Three-Phase PI Section Line2/RConn3 -- variable load 6/LConn3

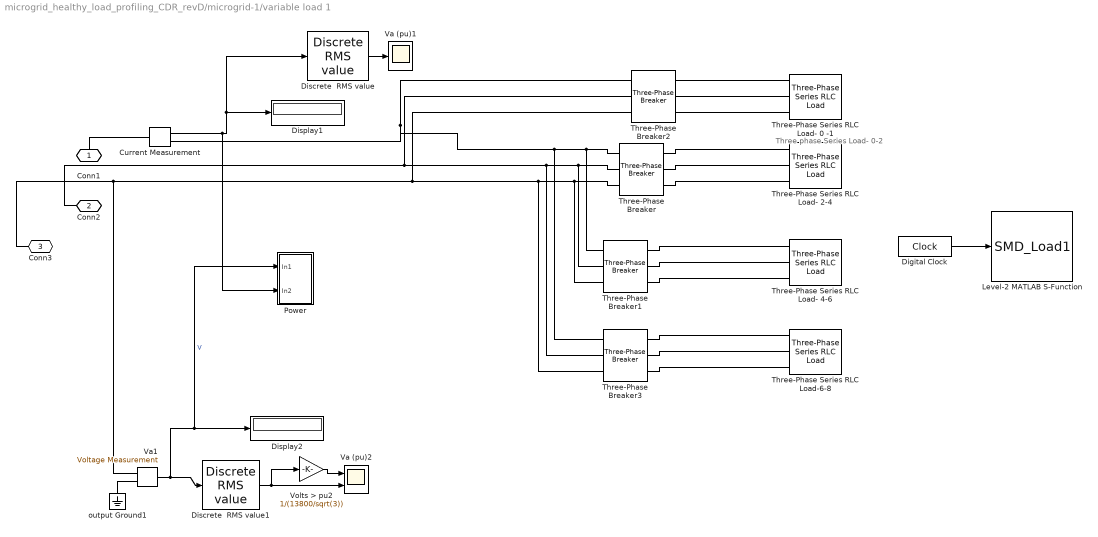
== system microgrid_healthy_load_profiling_CDR_revD/microgrid-1/variable load 1 ==
  note: Three phase Series Load- 0-2
  Current Measurement : powerlib/Measurements/Current Measurement  PhasorSimulation=off  OutputType=Complex  PSBequivalent=0
  Digital Clock : DigitalClock  SampleTime=Ts
  Discrete  RMS value : powerlib_extras/Discrete Measurements/Discrete  RMS value  Freq=60  Mag_Init=0  Ts=Ts
  Discrete  RMS value1 : powerlib_extras/Discrete Measurements/Discrete  RMS value  Freq=60  Mag_Init=0  Ts=Ts
  Display1 : Display
  Display2 : Display
  Level-2 MATLAB S-Function : M-S-Function  FunctionName=SMD_Load1  Parameters=tl1
  Power : Subsystem
  Three-Phase Series RLC Load- 0 -1 : powerlib/Elements/Three-Phase Series RLC Load  LConnTagsString=A|B|C  Configuration=Y (grounded)  NominalVoltage=13800  NominalFrequency=60  ActivePower=3.2e6  InductivePower=3.84e6  CapacitivePower=0  Measurements=None  LoadType=constant Z
  Three-Phase Series RLC Load- 2-4 : powerlib/Elements/Three-Phase Series RLC Load  LConnTagsString=A|B|C  Configuration=Y (grounded)  NominalVoltage=13800  NominalFrequency=60  ActivePower=4e6  InductivePower=3e6  CapacitivePower=0  Measurements=None  LoadType=constant Z
  Three-Phase Series RLC Load- 4-6 : powerlib/Elements/Three-Phase Series RLC Load  LConnTagsString=A|B|C  Configuration=Y (grounded)  NominalVoltage=13800  NominalFrequency=60  ActivePower=3.64e6  InductivePower=3.428e6  CapacitivePower=0  Measurements=None  LoadType=constant Z
  Three-Phase Series RLC Load-6-8 : powerlib/Elements/Three-Phase Series RLC Load  LConnTagsString=A|B|C  Configuration=Y (grounded)  NominalVoltage=13800  NominalFrequency=60  ActivePower=3.8e6  InductivePower=0  CapacitivePower=3.25e6  Measurements=None  LoadType=constant Z
  Three-Phase Breaker : powerlib/Elements/Three-Phase Breaker  InitialState=open  SwitchA=on  SwitchB=on  SwitchC=on  SwitchTimes=[tl1(1)/60 tl1(2)/60]  External=off  BreakerResistance=0.001  SnubberResistance=1e6  SnubberCapacitance=inf  Measurements=None
  Three-Phase Breaker1 : powerlib/Elements/Three-Phase Breaker  InitialState=open  SwitchA=on  SwitchB=on  SwitchC=on  SwitchTimes="[tl1(2)/60  tl1(3)/60]"  External=off  BreakerResistance=0.001  SnubberResistance=1e6  SnubberCapacitance=inf  Measurements=None
  Three-Phase Breaker2 : powerlib/Elements/Three-Phase Breaker  InitialState=closed  SwitchA=on  SwitchB=on  SwitchC=on  SwitchTimes=[tl1(1)/60]  External=off  BreakerResistance=0.001  SnubberResistance=1e6  SnubberCapacitance=inf  Measurements=None
  Three-Phase Breaker3 : powerlib/Elements/Three-Phase Breaker  InitialState=open  SwitchA=on  SwitchB=on  SwitchC=on  SwitchTimes=[tl1(3)/60]  External=off  BreakerResistance=0.001  SnubberResistance=1e6  SnubberCapacitance=inf  Measurements=None
  Va (pu)1 : Scope
      settings: TickLabels=on  TimeRange=2  YMin=128.764  YMax=128.764  SaveName=vf6
  Va (pu)2 : Scope  NumInputPorts=2
      settings: TickLabels=on  TimeRange=3  YMin=0~7153.5  YMax=2~7163.5  SaveName=vf2
  Va1 : powerlib/Measurements/Voltage Measurement  Tag=PoWeRsYsTeMmEaSuReMeNt  PhasorSimulation=off  OutputType=Magnitude  PSBequivalent=0
  Volts > pu2 : Gain  Gain=1/(13800/sqrt(3))  SaturateOnIntegerOverflow=on  OutDataTypeStr=Inherit: Same as input  ParamDataTypeStr=Inherit: Same as input
  output Ground1 : powerlib/Elements/Ground  LConnTagsString=a
  Conn1 : PMIOPort  Port=1  Side=Left
  Conn2 : PMIOPort  Port=2  Side=Left
  Conn3 : PMIOPort  Port=3  Side=Left
  wires:
  Va1/1 -> Display2/1, Power/1(In1), Discrete  RMS value1/1  "V"
  Current Measurement/1 -> Display1/1, Discrete  RMS value/1, Power/2(In2)
  Discrete  RMS value/1 -> Va (pu)1/1
  Discrete  RMS value1/1 -> Va (pu)2/2, Volts > pu2/1
  Volts > pu2/1 -> Va (pu)2/1
  Digital Clock/1 -> Level-2 MATLAB S-Function/1
  connections:
  Three-Phase Breaker/RConn1 -- Three-Phase Series RLC Load- 2-4/LConn1
  Three-Phase Breaker/RConn2 -- Three-Phase Series RLC Load- 2-4/LConn2
  Three-Phase Breaker/RConn3 -- Three-Phase Series RLC Load- 2-4/LConn3
  Three-Phase Breaker1/RConn1 -- Three-Phase Series RLC Load- 4-6/LConn1
  Three-Phase Breaker1/RConn2 -- Three-Phase Series RLC Load- 4-6/LConn2
  Three-Phase Breaker1/RConn3 -- Three-Phase Series RLC Load- 4-6/LConn3
  Three-Phase Breaker3/LConn1 -- Current Measurement/RConn1 -- Three-Phase Breaker2/LConn1 -- Three-Phase Breaker/LConn1 -- Three-Phase Breaker1/LConn1
  Three-Phase Breaker3/LConn2 -- Conn2/RConn1 -- Three-Phase Breaker2/LConn2 -- Three-Phase Breaker/LConn2 -- Three-Phase Breaker1/LConn2
  Three-Phase Breaker3/LConn3 -- Conn3/RConn1 -- Va1/LConn1 -- Three-Phase Breaker2/LConn3 -- Three-Phase Breaker/LConn3 -- Three-Phase Breaker1/LConn3
  Three-Phase Breaker2/RConn2 -- Three-Phase Series RLC Load- 0 -1/LConn2
  Three-Phase Breaker2/RConn3 -- Three-Phase Series RLC Load- 0 -1/LConn3
  output Ground1/LConn1 -- Va1/LConn2
  Conn1/RConn1 -- Current Measurement/LConn1
  Three-Phase Breaker2/RConn1 -- Three-Phase Series RLC Load- 0 -1/LConn1
  Three-Phase Breaker3/RConn1 -- Three-Phase Series RLC Load-6-8/LConn1
  Three-Phase Breaker3/RConn2 -- Three-Phase Series RLC Load-6-8/LConn2
  Three-Phase Breaker3/RConn3 -- Three-Phase Series RLC Load-6-8/LConn3

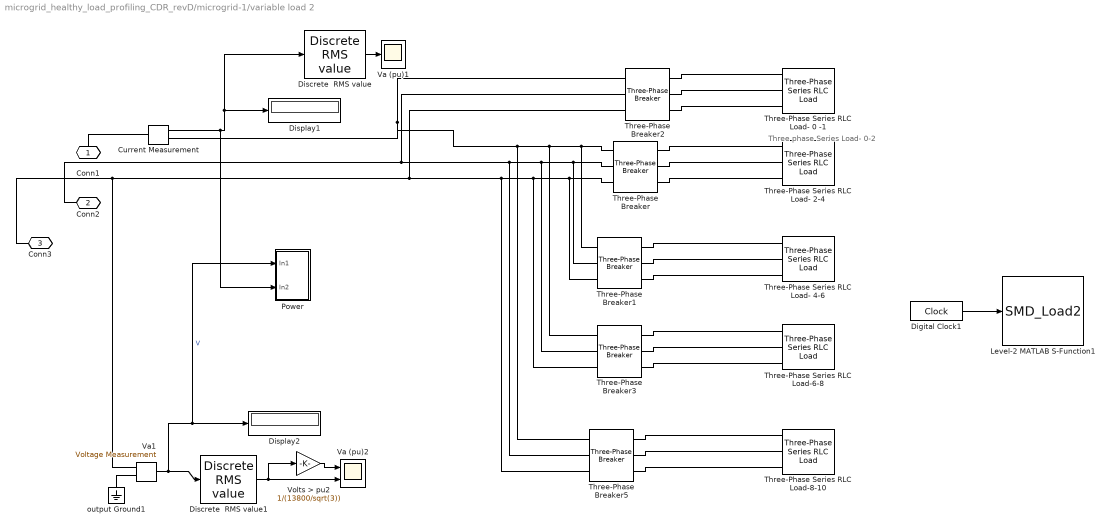
== system microgrid_healthy_load_profiling_CDR_revD/microgrid-1/variable load 2 ==
  note: Three phase Series Load- 0-2
  Current Measurement : powerlib/Measurements/Current Measurement  PhasorSimulation=off  OutputType=Complex  PSBequivalent=0
  Digital Clock1 : DigitalClock  SampleTime=Ts
  Discrete  RMS value : powerlib_extras/Discrete Measurements/Discrete  RMS value  Freq=60  Mag_Init=0  Ts=Ts
  Discrete  RMS value1 : powerlib_extras/Discrete Measurements/Discrete  RMS value  Freq=60  Mag_Init=0  Ts=Ts
  Display1 : Display
  Display2 : Display
  Level-2 MATLAB S-Function1 : M-S-Function  FunctionName=SMD_Load2  Parameters=tl2
  Power : Subsystem
  Three-Phase Series RLC Load- 0 -1 : powerlib/Elements/Three-Phase Series RLC Load  LConnTagsString=A|B|C  Configuration=Y (grounded)  NominalVoltage=13800  NominalFrequency=60  ActivePower=3.6e6  InductivePower=0  CapacitivePower=3.47e6  Measurements=None  LoadType=constant Z
  Three-Phase Series RLC Load- 2-4 : powerlib/Elements/Three-Phase Series RLC Load  LConnTagsString=A|B|C  Configuration=Y (grounded)  NominalVoltage=13800  NominalFrequency=60  ActivePower=2e6  InductivePower=4.27e6  CapacitivePower=0  Measurements=None  LoadType=constant Z
  Three-Phase Series RLC Load- 4-6 : powerlib/Elements/Three-Phase Series RLC Load  LConnTagsString=A|B|C  Configuration=Y (grounded)  NominalVoltage=13800  NominalFrequency=60  ActivePower=3e6  InductivePower=0  CapacitivePower=4e6  Measurements=None  LoadType=constant Z
  Three-Phase Series RLC Load-6-8 : powerlib/Elements/Three-Phase Series RLC Load  LConnTagsString=A|B|C  Configuration=Y (grounded)  NominalVoltage=13800  NominalFrequency=60  ActivePower=3.4e6  InductivePower=3.67e6  CapacitivePower=0  Measurements=None  LoadType=constant Z
  Three-Phase Series RLC Load-8-10 : powerlib/Elements/Three-Phase Series RLC Load  LConnTagsString=A|B|C  Configuration=Y (grounded)  NominalVoltage=13800  NominalFrequency=60  ActivePower=3.8e6  InductivePower=3.25e6  CapacitivePower=0  Measurements=None  LoadType=constant Z
  Three-Phase Breaker : powerlib/Elements/Three-Phase Breaker  InitialState=open  SwitchA=on  SwitchB=on  SwitchC=on  SwitchTimes=[tl2(1)/60 tl2(2)/60]  External=off  BreakerResistance=0.001  SnubberResistance=1e6  SnubberCapacitance=inf  Measurements=None
  Three-Phase Breaker1 : powerlib/Elements/Three-Phase Breaker  InitialState=open  SwitchA=on  SwitchB=on  SwitchC=on  SwitchTimes="[tl2(2)/60  tl2(3)/60]"  External=off  BreakerResistance=0.001  SnubberResistance=1e6  SnubberCapacitance=inf  Measurements=None
  Three-Phase Breaker2 : powerlib/Elements/Three-Phase Breaker  InitialState=closed  SwitchA=on  SwitchB=on  SwitchC=on  SwitchTimes=[tl2(1)/60]  External=off  BreakerResistance=0.001  SnubberResistance=1e6  SnubberCapacitance=inf  Measurements=None
  Three-Phase Breaker3 : powerlib/Elements/Three-Phase Breaker  InitialState=open  SwitchA=on  SwitchB=on  SwitchC=on  SwitchTimes="[tl2(3)/60  tl2(4)/60]"  External=off  BreakerResistance=0.001  SnubberResistance=1e6  SnubberCapacitance=inf  Measurements=None
  Three-Phase Breaker5 : powerlib/Elements/Three-Phase Breaker  InitialState=open  SwitchA=on  SwitchB=on  SwitchC=on  SwitchTimes=[tl2(4)/60 ]  External=off  BreakerResistance=0.001  SnubberResistance=1e6  SnubberCapacitance=inf  Measurements=None
  Va (pu)1 : Scope
      settings: TickLabels=on  TimeRange=2  YMin=-0.8  YMax=0.8  SaveName=vf6
  Va (pu)2 : Scope  NumInputPorts=2
      settings: TickLabels=on  TimeRange=3  YMin=0.8979~7153.5  YMax=0.8991~7163.5  SaveName=vf2
  Va1 : powerlib/Measurements/Voltage Measurement  Tag=PoWeRsYsTeMmEaSuReMeNt  PhasorSimulation=off  OutputType=Magnitude  PSBequivalent=0
  Volts > pu2 : Gain  Gain=1/(13800/sqrt(3))  SaturateOnIntegerOverflow=on  OutDataTypeStr=Inherit: Same as input  ParamDataTypeStr=Inherit: Same as input
  output Ground1 : powerlib/Elements/Ground  LConnTagsString=a
  Conn1 : PMIOPort  Port=1  Side=Left
  Conn2 : PMIOPort  Port=2  Side=Left
  Conn3 : PMIOPort  Port=3  Side=Left
  wires:
  Volts > pu2/1 -> Va (pu)2/1
  Discrete  RMS value1/1 -> Volts > pu2/1, Va (pu)2/2
  Discrete  RMS value/1 -> Va (pu)1/1
  Current Measurement/1 -> Power/2(In2), Display1/1, Discrete  RMS value/1
  Va1/1 -> Discrete  RMS value1/1, Power/1(In1), Display2/1  "V"
  Digital Clock1/1 -> Level-2 MATLAB S-Function1/1
  connections:
  Three-Phase Breaker5/RConn3 -- Three-Phase Series RLC Load-8-10/LConn3
  Three-Phase Breaker5/RConn2 -- Three-Phase Series RLC Load-8-10/LConn2
  Three-Phase Breaker5/RConn1 -- Three-Phase Series RLC Load-8-10/LConn1
  Three-Phase Breaker3/RConn3 -- Three-Phase Series RLC Load-6-8/LConn3
  Three-Phase Breaker3/RConn2 -- Three-Phase Series RLC Load-6-8/LConn2
  Three-Phase Breaker3/RConn1 -- Three-Phase Series RLC Load-6-8/LConn1
  Three-Phase Breaker2/RConn1 -- Three-Phase Series RLC Load- 0 -1/LConn1
  Conn1/RConn1 -- Current Measurement/LConn1
  output Ground1/LConn1 -- Va1/LConn2
  Three-Phase Breaker2/RConn3 -- Three-Phase Series RLC Load- 0 -1/LConn3
  Three-Phase Breaker2/RConn2 -- Three-Phase Series RLC Load- 0 -1/LConn2
  Three-Phase Breaker3/LConn3 -- Three-Phase Breaker1/LConn3 -- Three-Phase Breaker/LConn3 -- Three-Phase Breaker2/LConn3 -- Va1/LConn1 -- Conn3/RConn1 -- Three-Phase Breaker5/LConn3
  Three-Phase Breaker3/LConn2 -- Three-Phase Breaker1/LConn2 -- Three-Phase Breaker/LConn2 -- Three-Phase Breaker2/LConn2 -- Conn2/RConn1 -- Three-Phase Breaker5/LConn2
  Three-Phase Breaker3/LConn1 -- Three-Phase Breaker1/LConn1 -- Three-Phase Breaker/LConn1 -- Three-Phase Breaker2/LConn1 -- Current Measurement/RConn1 -- Three-Phase Breaker5/LConn1
  Three-Phase Breaker1/RConn3 -- Three-Phase Series RLC Load- 4-6/LConn3
  Three-Phase Breaker1/RConn2 -- Three-Phase Series RLC Load- 4-6/LConn2
  Three-Phase Breaker1/RConn1 -- Three-Phase Series RLC Load- 4-6/LConn1
  Three-Phase Breaker/RConn3 -- Three-Phase Series RLC Load- 2-4/LConn3
  Three-Phase Breaker/RConn2 -- Three-Phase Series RLC Load- 2-4/LConn2
  Three-Phase Breaker/RConn1 -- Three-Phase Series RLC Load- 2-4/LConn1

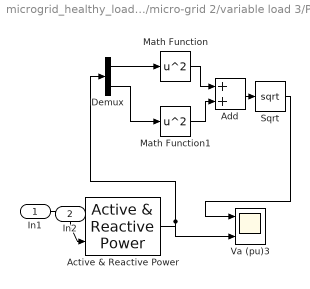
== system microgrid_healthy_load_profiling_CDR_revD/micro-grid 2/variable load 3/Power ==
  In1 : Inport
  In2 : Inport  Port=2
  Active & Reactive Power : powerlib_extras/Measurements/Active & Reactive Power  f1=60
  Add : Sum
  Demux : Demux  Outputs=2
  Math Function : Math  Operator=square  OutputSignalType=real  SaturateOnIntegerOverflow=on
  Math Function1 : Math  Operator=square  OutputSignalType=real  SaturateOnIntegerOverflow=on
  Sqrt : Sqrt  SaturateOnIntegerOverflow=on
  Va (pu)3 : Scope  NumInputPorts=2
      settings: TickLabels=on  TimeRange=2  YMin=206676~-125000  YMax=206700~175000  SaveName=vf3
  wires:
  In2/1 -> Active & Reactive Power/2
  In1/1 -> Active & Reactive Power/1
  Sqrt/1 -> Va (pu)3/1
  Add/1 -> Sqrt/1
  Math Function1/1 -> Add/2
  Demux/2 -> Math Function1/1
  Math Function/1 -> Add/1
  Demux/1 -> Math Function/1
  Active & Reactive Power/1 -> Va (pu)3/2, Demux/1

== system microgrid_healthy_load_profiling_CDR_revD/micro-grid 2/variable load 4/Power ==
  In1 : Inport
  In2 : Inport  Port=2
  Active & Reactive Power : powerlib_extras/Measurements/Active & Reactive Power  f1=60
  Add : Sum
  Demux : Demux  Outputs=2
  Math Function : Math  Operator=square  OutputSignalType=real  SaturateOnIntegerOverflow=on
  Math Function1 : Math  Operator=square  OutputSignalType=real  SaturateOnIntegerOverflow=on
  Sqrt : Sqrt  SaturateOnIntegerOverflow=on
  Va (pu)3 : Scope  NumInputPorts=2
      settings: TickLabels=on  TimeRange=2  YMin=206676~-125000  YMax=206700~175000  SaveName=vf3
  wires:
  Active & Reactive Power/1 -> Demux/1, Va (pu)3/2
  Demux/1 -> Math Function/1
  Math Function/1 -> Add/1
  Demux/2 -> Math Function1/1
  Math Function1/1 -> Add/2
  Add/1 -> Sqrt/1
  Sqrt/1 -> Va (pu)3/1
  In1/1 -> Active & Reactive Power/1
  In2/1 -> Active & Reactive Power/2
